simulink model "Sistema_Nonlineare"  (R2020b)
settings: Solver=VariableStepAuto  StartTime=0.0  StopTime=100  RelTol=1e-3
settings Model: Creator=Stefano  LastModifiedBy=Stefano

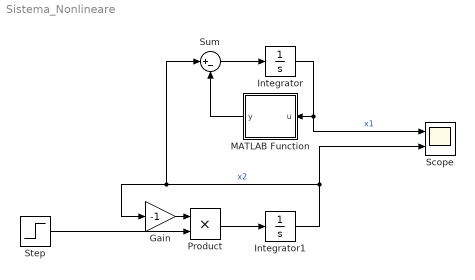
== system Sistema_Nonlineare ==
  Gain : Gain  Gain=-1
  Integrator : Integrator  InitialCondition=1
  Integrator1 : Integrator  InitialCondition=1
  MATLAB Function : MATLAB Function  TreatAsAtomicUnit=on
  Product : Product
  Scope : Scope  NumInputPorts=2
  Step : Step  SampleTime=0
  Sum : Sum  Inputs=|+-
  wires:
  Integrator/1 -> Scope/1, MATLAB Function/1(u)  "x1"
  Integrator1/1 -> Scope/2, Gain/1, Sum/1  "x2"
  MATLAB Function/1(y) -> Sum/2
  Sum/1 -> Integrator/1
  Product/1 -> Integrator1/1
  Step/1 -> Product/2
  Gain/1 -> Product/1

== matlab function Sistema_Nonlineare/MATLAB Function ==
  data: u input; y output
function y = quadrato(u)

y = u^2;
